simulink model "rocket"  (R2023a)
settings: Solver=ode3  StartTime=0.0  StopTime=Tf  FixedStep=dt  MaxStep=0.05  RelTol=1e-3  EnableMultiTasking=on
undefined symbols (not defined in the file or in its folder): alpha0, d2r, delta0, mach0, q0
settings Model: Creator=pjseiler  LastModifiedBy=jdlarson1
settings SolverCC: AlgebraicLoopSolver=TrustRegion
settings DataIOCC: LimitDataPoints=on  SaveFormat=Array  SignalLoggingSaveFormat=ModelDataLogs  ReturnWorkspaceOutputs=off
settings OptimizationCC: ReuseModelBlockBuffer=off  ExpressionDepthLimit=2147483647  LifeSpan=inf
settings DebuggingCC: UnderspecifiedInitializationDetection=Classic  MergeDetectMultiDrivingBlocksExec=none  SolverPrmCheckMsg=warning  FcnCallInpInsideContextMsg=warning  UnconnectedInputMsg=warning  UnconnectedOutputMsg=warning  UnconnectedLineMsg=warning  StateNameClashWarn=warning  SFUnexpectedBacktrackingDiag=warning  SFNoUnconditionalDefaultTransitionDiag=warning  SFExecutionAtInitializationDiag=none  ArithmeticOperatorsInVariantConditions=warning
settings HardwareCC: ProdBitPerPointer=32  ProdBitPerSizeT=32  ProdBitPerPtrDiffT=32  ProdLargestAtomicFloat=None  ProdIntDivRoundTo=Undefined  ProdEndianess=Unspecified  ProdWordSize=32  ProdHWDeviceType=32-bit Generic
settings ModelReferenceCC: PropagateSignalLabelsOutOfModel=off
settings SFSimCC: SimUseLocalCustomCode=off  CustomCodeUndefinedFunction=UseInterfaceOnly
settings RTWCC: RTWUseLocalCustomCode=off
settings CodeAppCC: StateflowObjectComments=on
settings GRTTargetCC: TargetLangStandard=C89/C90 (ANSI)  CombineOutputUpdateFcns=off  GRTInterface=on
settings ConfigComp: CovMetricSettings=dw  CovSaveCumulativeToWorkspaceVar=on  CovSaveSingleToWorkspaceVar=on  CovExternalEMLEnable=off

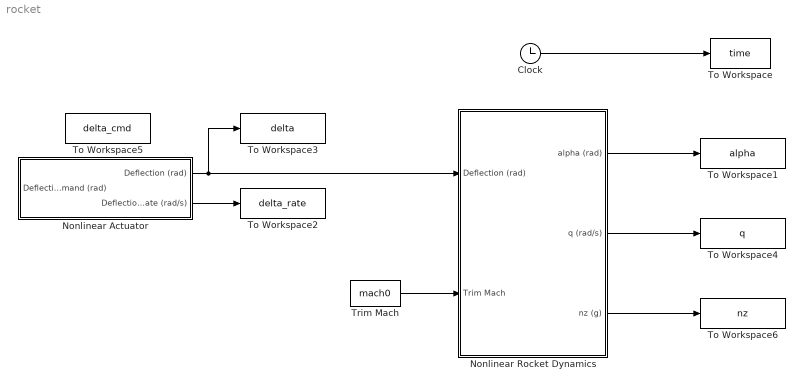
== system rocket ==
  Clock : Clock
  Nonlinear Actuator : Subsystem
  Nonlinear Rocket Dynamics : Subsystem
  To Workspace : ToWorkspace  VariableName=time  SampleTime=-1
  To Workspace1 : ToWorkspace  VariableName=alpha  SampleTime=-1
  To Workspace2 : ToWorkspace  VariableName=delta_rate  SampleTime=-1
  To Workspace3 : ToWorkspace  VariableName=delta  SampleTime=-1
  To Workspace4 : ToWorkspace  VariableName=q  SampleTime=-1
  To Workspace5 : ToWorkspace  VariableName=delta_cmd  SampleTime=-1
  To Workspace6 : ToWorkspace  VariableName=nz  SampleTime=-1
  Trim Mach : Constant  Value=mach0
  wires:
  Nonlinear Actuator/1(Deflection (rad)) -> Nonlinear Rocket Dynamics/1(Deflection (rad)), To Workspace3/1
  Clock/1 -> To Workspace/1
  Nonlinear Actuator/2(Deflection Rate (rad/s)) -> To Workspace2/1
  Trim Mach/1 -> Nonlinear Rocket Dynamics/2(Trim Mach)
  Nonlinear Rocket Dynamics/2(q (rad/s)) -> To Workspace4/1
  Nonlinear Rocket Dynamics/3(nz (g)) -> To Workspace6/1
  Nonlinear Rocket Dynamics/1(alpha (rad)) -> To Workspace1/1
  ? -> To Workspace5/1, Nonlinear Actuator/1(Deflection command (rad))

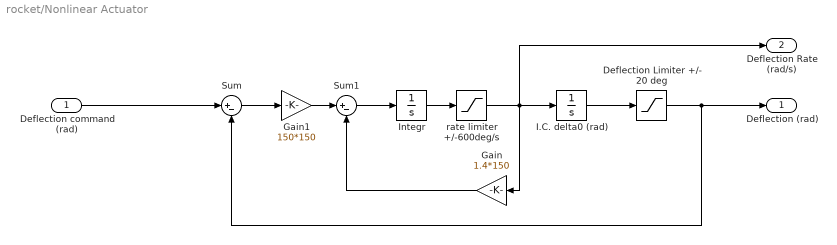
== system rocket/Nonlinear Actuator ==
  Deflection command (rad) : Inport
  Deflection Limiter +/- 20 deg : Saturate  UpperLimit=20*d2r  LowerLimit=-20*d2r
  Gain : Gain  Gain=1.4*150
  Gain1 : Gain  Gain=150*150
  I.C. delta0 (rad) : Integrator  InitialCondition=delta0
  Integr : Integrator
  Sum : Sum  Inputs=|+-
  Sum1 : Sum  Inputs=|+-
  rate limiter +/-600deg/s : Saturate  UpperLimit=600*d2r  LowerLimit=-600*d2r
  Deflection (rad) : Outport
  Deflection Rate (rad/s) : Outport  Port=2
  wires:
  Integr/1 -> rate limiter +/-600deg/s/1
  Deflection command (rad)/1 -> Sum/1
  Sum1/1 -> Integr/1
  Gain/1 -> Sum1/2
  Gain1/1 -> Sum1/1
  rate limiter +/-600deg/s/1 -> I.C. delta0 (rad)/1, Deflection Rate (rad/s)/1, Gain/1
  Deflection Limiter +/- 20 deg/1 -> Deflection (rad)/1, Sum/2
  I.C. delta0 (rad)/1 -> Deflection Limiter +/- 20 deg/1
  Sum/1 -> Gain1/1

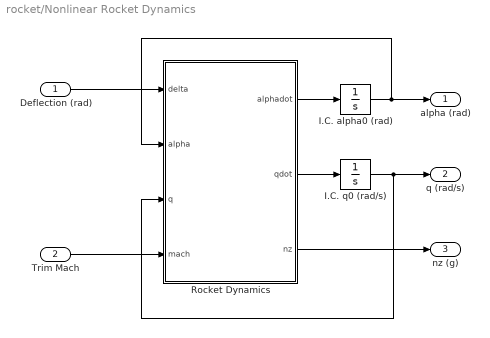
== system rocket/Nonlinear Rocket Dynamics ==
  Deflection (rad) : Inport
  Trim Mach : Inport  Port=2
  I.C. alpha0 (rad) : Integrator  InitialCondition=alpha0
  I.C. q0 (rad/s) : Integrator  InitialCondition=q0
  Rocket Dynamics : MATLAB Function  TreatAsAtomicUnit=on
  alpha (rad) : Outport
  q (rad/s) : Outport  Port=2
  nz (g) : Outport  Port=3
  wires:
  Rocket Dynamics/3(nz) -> nz (g)/1
  I.C. alpha0 (rad)/1 -> Rocket Dynamics/2(alpha), alpha (rad)/1
  I.C. q0 (rad/s)/1 -> q (rad/s)/1, Rocket Dynamics/3(q)
  Deflection (rad)/1 -> Rocket Dynamics/1(delta)
  Trim Mach/1 -> Rocket Dynamics/4(mach)
  Rocket Dynamics/1(alphadot) -> I.C. alpha0 (rad)/1
  Rocket Dynamics/2(qdot) -> I.C. q0 (rad/s)/1

== matlab function rocket/Nonlinear Rocket Dynamics/Rocket Dynamics ==
  data: delta input; alpha input; q input; alphadot output; qdot output; nz output; mach input
function [alphadot, qdot, nz] = rocket_dynamics(delta, alpha, q, mach)

% Unit conversion factors
d2r = pi/180;               % Degrees to radians
r2d = 1/d2r;                % Radians to degrees

% Aircraft Parameters
p_s = 973.3;         % Static pressure at 20000ft, lbs/ft^2
c_s = 1036.4;        % Speed of sound at 20000ft, ft/sec
S_ref = 0.44;        % Reference area, ft^2
d = 0.75;            % Diameter, ft
mass = 13.98;        % Mass, slugs
inertia_y = 182.5;   % Pitch moment of inertia, slug*ft^2
gravity = 32.2;      % Gravitational acceleration, ft/sec^2

% Aerodynamic coefficients for Cn and Cm: See project file for more
% details. The coefficients n1 and m1 depend on Mach number as:
%   n1 = n1a+n1b*Mach
%   m1 = m1a+m1b*Mach
n0= -0.034*r2d; 
n2= -9.4457e-3*r2d^2; 
n3 = 0.000103*r2d^3;
m0= -0.206*r2d; 
m2= -1.9546e-2*r2d^2;
m3 = 0.000215*r2d^3;

n1a = -2*0.1696*r2d;
n1b = 0.1696/3*r2d;

m1a =  -7*0.051*r2d;
m1b =  8/3*0.051*r2d;

% Dynamic pressure and airspeed
dynamic_pressure = 0.7*p_s*mach^2;

% Remaining aero coefficients at specified Mach number
n1 = n1a+n1b*mach;
m1 = m1a+m1b*mach;

% Aerodynamic Forces
force_coef = sign(alpha)*(n3*abs(alpha)^3 + n2*alpha^2 + ...
    n1*abs(alpha)) + n0*delta;
moment_coef = sign(alpha)*(m3*abs(alpha)^3 + m2*alpha^2 + ...
    m1*abs(alpha)) + m0*delta;
vertical_force = force_coef*dynamic_pressure*S_ref;
y_moment = moment_coef *dynamic_pressure*S_ref*d;

% compute alphadot and qdot vector
alphadot = cos(alpha)*vertical_force/(mass*mach*c_s) + q;
qdot = y_moment/inertia_y;
nz = d2r*vertical_force/(mass*gravity);
